simulink model "nonlinearSim"  (Simulink 8.3)
settings: Solver=ode45  StartTime=0.0  StopTime=20  MaxStep=0.01  RelTol=1e-3
settings Model: Creator=shahin  LastModifiedBy=shiv
settings OptimizationCC: ExpressionDepthLimit=2147483647
settings DebuggingCC: FcnCallInpInsideContextMsg=EnableAllAsWarning

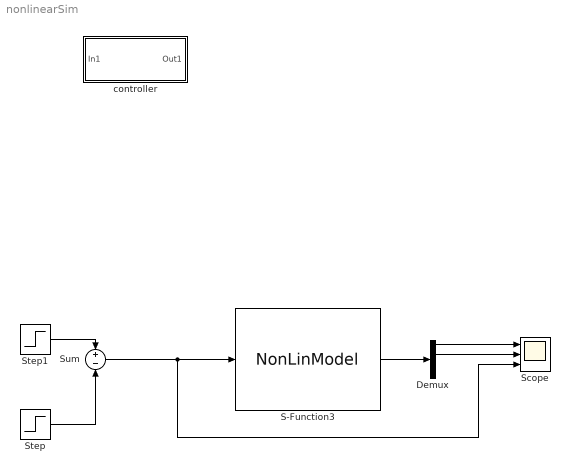
== system nonlinearSim ==
  Demux : Demux
  S-Function3 : S-Function  FunctionName=NonLinModel  Parameters=[pi/2,0,0,0],[10.1215 0.3972 0.1035 6.3513 1.2253 39.3578 0.0042]  EnableBusSupport=off
  Scope : Scope  NumInputPorts=3
      settings: TickLabels=on  YMin=0.5~-5~-5  YMax=2.7~5~5
  Step : Step  Time=3.1  After=0.1  SampleTime=0
  Step1 : Step  Time=3  After=0.1  SampleTime=0
  Sum : Sum  Inputs=+-
  controller : Subsystem
  wires:
  S-Function3/1 -> Demux/1
  Demux/1 -> Scope/1
  Demux/2 -> Scope/2
  Step/1 -> Sum/2
  Step1/1 -> Sum/1
  Sum/1 -> Scope/3, S-Function3/1

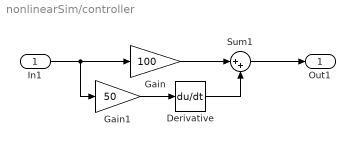
== system nonlinearSim/controller ==
  In1 : Inport
  Derivative : Derivative
  Gain : Gain  Gain=100
  Gain1 : Gain  Gain=50
  Sum1 : Sum  Inputs=|++
  Out1 : Outport
  wires:
  Gain1/1 -> Derivative/1
  In1/1 -> Gain1/1, Gain/1
  Derivative/1 -> Sum1/2
  Gain/1 -> Sum1/1
  Sum1/1 -> Out1/1
